simulink model "VDP3"  (R2017b)
settings: Solver=FixedStepAuto  StartTime=0.0  StopTime=1  FixedStep=0.005  RelTol=1e-3
values from neighbouring files (symbols this model uses):
  mu = 5    [VDP_mainc.m]
  tF = yF(end)    [VDP_mainc.m]
settings Model: Creator=Soutrik  LastModifiedBy=Soutrik

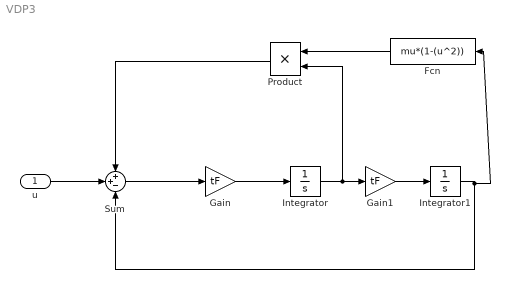
== system VDP3 ==
  u : Inport
  Fcn : Fcn  Expr=mu*(1-(u^2))
  Gain : Gain  Gain=tF
  Gain1 : Gain  Gain=tF
  Integrator : Integrator
  Integrator1 : Integrator
  Product : Product
  Sum : Sum  Inputs=++-
  wires:
  Gain/1 -> Integrator/1
  Gain1/1 -> Integrator1/1
  Integrator/1 -> Product/2, Gain1/1
  Sum/1 -> Gain/1
  Integrator1/1 -> Fcn/1, Sum/3
  Product/1 -> Sum/1
  u/1 -> Sum/2
  Fcn/1 -> Product/1
